simulink model "sheme"  (R2017b)
settings: Solver=VariableStepAuto  StartTime=0.0  StopTime=15  MaxStep=0.01  RelTol=1e-3
InitFcn:
  | % éÓÈÏÄÎÙÅ ÄÁÎÎÙÅ
  | A=[0 5/4; 1 6/4]
  | B=[-1; 3/4]
  | C=[0 1]
  | Bf=[-2; 5/4];
  | 
  | % òÁÓÛÉÒÅÎÎÁÑ ÍÏÄÅÌØ ÏÛÉÂÏË
  | G=[1;0];
  | Ge=[1;0];
  | Gamma_f=[0 1;-81 0];
  | H_f=[1 0];
  | Gamma_g=[0 1;-4 0];
  | H_g=[1 0];
  | A_bar=[Gamma_f zeros(2,2) G*C; zeros(2,2) Gamma_g -Ge*C; zeros(2,4) A];
  | B_bar=[zeros(4,1); B];
  | 
  | % ÷ÙÞÉÓÌÅÎÉÅ ÍÁÔÒÉÃÙ ÌÉÎÅÊÎÙÈ ÓÔÁÃÉÏÎÁÒÎÙÈ ÏÂÒÁÔÎÙÈ Ó×ÑÚÅÊ
  | Gamma_bar=[-5.2 1 0 0 0 0;
  |            -1 -5.2 1 0 0 0;
  |            0 0 -5.1 1 0 0;
  |            0 0 0 -5.9 1 0;
  |            0 0 0 0 -5.8 1;
  |            0 0 0 0 0 -5.5];
  | H_bar=[1 0 1 1 1 1];
  | M_bar=sylv(-A_bar, Gamma_bar, B_bar*H_bar);
  | K_bar=-H_bar*inv(M_bar)
  | 
  | %îÁÂÌÀÄÁÔÅÌØ
  | Gamma=[-5.25 0; 0 -5.95];
  | H=[1 1];
  | M=sylv(-A', Gamma, C'*H);
  | L=(-H*inv(M))';
settings Model: Creator=lida  LastModifiedBy=lida

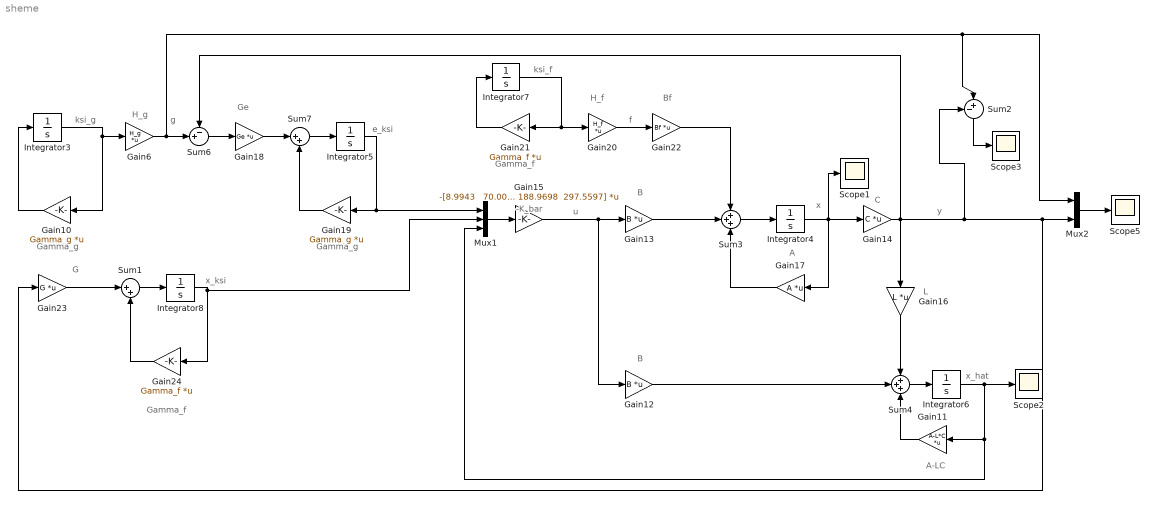
== system sheme ==
  note: L
  note: A
  note: Ge
  note: A-LC
  note: B
  note: Gamma_g
  note: B
  note: x_hat
  note: H_g
  note: -K_bar
  note: u
  note: Gamma_g
  note: y
  note: C
  note: ksi_g
  note: e_ksi
  note: x
  note: g
  note: Bf
  note: H_f
  note: f
  note: Gamma_f
  note: ksi_f
  note: x_ksi
  note: G
  note: Gamma_f
  Gain10 : Gain  Gain=Gamma_g  Multiplication=Matrix(K*u)
  Gain11 : Gain  Gain=A-L*C  Multiplication=Matrix(K*u)
  Gain12 : Gain  Gain=B  Multiplication=Matrix(K*u)
  Gain13 : Gain  Gain=B  Multiplication=Matrix(K*u)
  Gain14 : Gain  Gain=C  Multiplication=Matrix(K*u)
  Gain15 : Gain  Gain="-[8.9943   70.0091 274.9221   -8.7247 188.9698  297.5597]"  Multiplication=Matrix(K*u)
  Gain16 : Gain  Gain=L  Multiplication=Matrix(K*u)
  Gain17 : Gain  Gain=A  Multiplication=Matrix(K*u)
  Gain18 : Gain  Gain=Ge  Multiplication=Matrix(K*u)
  Gain19 : Gain  Gain=Gamma_g  Multiplication=Matrix(K*u)
  Gain20 : Gain  Gain=H_f  Multiplication=Matrix(K*u)
  Gain21 : Gain  Gain=Gamma_f  Multiplication=Matrix(K*u)
  Gain22 : Gain  Gain=Bf  Multiplication=Matrix(K*u)
  Gain23 : Gain  Gain=G  Multiplication=Matrix(K*u)
  Gain24 : Gain  Gain=Gamma_f  Multiplication=Matrix(K*u)
  Gain6 : Gain  Gain=H_g  Multiplication=Matrix(K*u)
  Integrator3 : Integrator  InitialCondition=[5*sin(-3); 10*cos(-3)]
  Integrator4 : Integrator  InitialCondition=[1;1]
  Integrator5 : Integrator  InitialCondition=[0;0]
  Integrator6 : Integrator
  Integrator7 : Integrator  InitialCondition=[3*cos(2);-27*sin(2)]
  Integrator8 : Integrator  InitialCondition=[0;0]
  Mux1 : Mux  Inputs=3
  Mux2 : Mux  Inputs=2
  Scope{1..3,5} (4 alike) : Scope
  Sum1 : Sum  Inputs=|++
  Sum2 : Sum  Inputs=-+|
  Sum3 : Sum  Inputs=+++
  Sum4 : Sum  Inputs=+++
  Sum6 : Sum  Inputs=-+|
  Sum7 : Sum  Inputs=|++
  wires:
  Integrator3/1 -> Gain10/1, Gain6/1
  Sum7/1 -> Integrator5/1
  Gain14/1 -> Sum6/1, Sum2/1, Gain23/1, Mux2/2, Gain16/1
  Integrator4/1 -> Scope1/1, Gain17/1, Gain14/1
  Gain12/1 -> Sum4/2
  Gain19/1 -> Sum7/2
  Gain10/1 -> Integrator3/1
  Gain15/1 -> Gain12/1, Gain13/1
  Mux1/1 -> Gain15/1
  Integrator5/1 -> Mux1/1, Gain19/1
  Sum4/1 -> Integrator6/1
  Gain16/1 -> Sum4/1
  Sum3/1 -> Integrator4/1
  Gain6/1 -> Sum2/2, Mux2/1, Sum6/2
  Integrator6/1 -> Scope2/1, Mux1/3, Gain11/1
  Gain18/1 -> Sum7/1
  Gain11/1 -> Sum4/3
  Sum6/1 -> Gain18/1
  Mux2/1 -> Scope5/1
  Gain17/1 -> Sum3/3
  Gain13/1 -> Sum3/2
  Gain21/1 -> Integrator7/1
  Integrator7/1 -> Gain21/1, Gain20/1
  Gain20/1 -> Gain22/1
  Gain22/1 -> Sum3/1
  Gain24/1 -> Sum1/2
  Sum1/1 -> Integrator8/1
  Integrator8/1 -> Mux1/2, Gain24/1
  Gain23/1 -> Sum1/1
  Sum2/1 -> Scope3/1
